simulink subsystem "StreetLaneSegment2x2_BUS_asSubsystem"  (R2021a)
settings: Solver=VariableStepAuto  StartTime=0.0  StopTime=10.0  RelTol=1e-3
undefined symbols (not defined in the file): x0z, xz, yin, yout, yz
libraries: StreetLanesLibrary x1
settings Model: Creator=phill  LastModifiedBy=phill

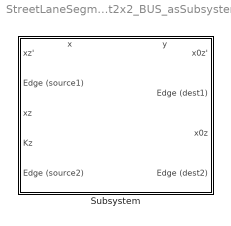
== system StreetLaneSegment2x2_BUS_asSubsystem ==
  Subsystem : Subsystem  mask{Kz=0, Tz=0}
      mask prompts: Kz "Kz (Capacity - How many cars fit into this cell)"; Tz "Tz (Nominal travel time for vehicles traveling unobstructed through the cell)"
      mask help: The 2x2 extension to the basic cell.
      settings: PortSchema="{\"entries\":[{\"content\":{\"sides\":[{\"content\":{\"connectorIds\":[\"Out5\",\"In1\",\"Out6\",\"Out7\",\"In2\"]},\"type\":\"ConnectorPlacement.EquallySpacedRectSide\",\"uuid\":\"0d72bc7f-f65e-4e07-ad8f-8c66e41d5ec5\"},{\"content\":{\"connectorIds\":[\"Out1\",\"In3\",\"Out2\",\"In4\"],\"side\":\"RIGHT\"},\"type\":\"ConnectorPlacement.EquallySpacedRectSide\",\"uuid\":\"af462cdf-0fa0-460f-8030-ea00e806c044\"},{\"content\":{\"connectorIds\":[\"Out3\",\"Out4\"],\"side\":\"TOP\"},\"type\":\"ConnectorPlacement.EquallySpacedRectSide\",\"uuid\":\"2548bddb-6962-4693-916e-1100869f2661\"}]},\"type\":\"ConnectorPlacement.EquallySpacedConnector\",\"uuid\":\"37811e3d-8b76-462d-b137-4aea1b95b5f4\"}],\"packageUris\":[\"http://schema.mathworks.com/mf0/Connector/R2020b\"],\"version\":\"1.0\"}"
      mask Display:
      | image('$imagefile'); % Use "Edit Image" on toolstrip to change.
      | disp('Street Lane Segment 2x2 \n\n');
      | disp(['Kz = ', get_param(gcb,'Kz'), ' | Tz = ', get_param(gcb, 'Tz')])

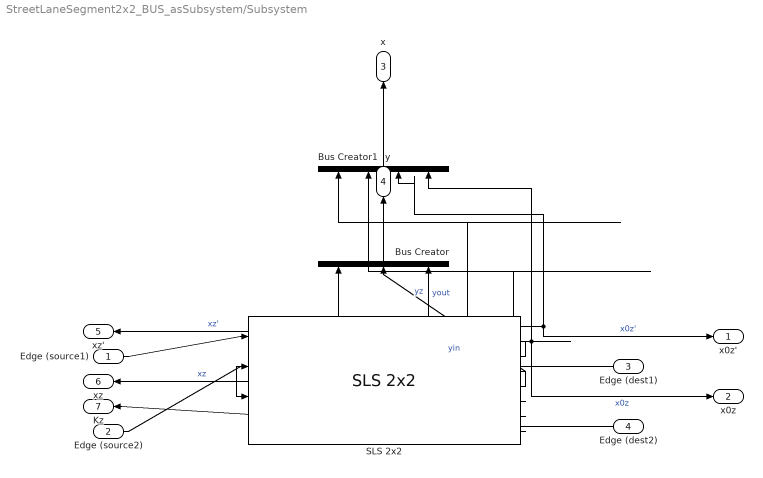
== system StreetLaneSegment2x2_BUS_asSubsystem/Subsystem ==
  Edge (source1) : Inport
  Edge (source2) : Inport  Port=2
  Edge (dest1) : Inport  Port=3
  Edge (dest2) : Inport  Port=4
  Bus Creator : BusCreator  Inputs=yin,yz,yout
  Bus Creator1 : BusCreator  Inputs=xz,xz',x0z',x0z
  SLS 2x2 : StreetLanesLibrary/SLS 2x2  Kz=0  Tz=0
  x0z' : Outport
  x0z : Outport  Port=2
  x : Outport  Port=3
  y : Outport  Port=4
  xz' : Outport  Port=5
  xz : Outport  Port=6
  Kz : Outport  Port=7
  wires:
  Bus Creator/1 -> y/1
  SLS 2x2/8 -> Kz/1
  SLS 2x2/6 -> xz'/1, Bus Creator1/2  "xz'"
  Bus Creator1/1 -> x/1
  SLS 2x2/1 -> x0z'/1, Bus Creator1/3  "x0z'"
  SLS 2x2/7 -> xz/1, Bus Creator1/1  "xz"
  SLS 2x2/2 -> x0z/1, Bus Creator1/4  "x0z"
  SLS 2x2/5 -> Bus Creator/3  "yout"
  SLS 2x2/4 -> Bus Creator/2  "yz"
  SLS 2x2/3 -> Bus Creator/1  "yin"
  Edge (source1)/1 -> SLS 2x2/1
  Edge (dest1)/1 -> SLS 2x2/3
  Edge (dest2)/1 -> SLS 2x2/4
  Edge (source2)/1 -> SLS 2x2/2
